simulink model "SISO_simulink_model"  (R2022a)
settings: Solver=VariableStepAuto  StartTime=0.0  StopTime=3  RelTol=1e-3
model workspace (MAT data in the model file):
  C = Simulink.Parameter
  C.Value = 525.1
  C.DataType = 'auto'
  C.Complexity = 'real'
  C.Dimensions = [1 1]
  D = Simulink.Parameter
  D.Value = 0.6069
  D.Description = 'Damping EFE'
  D.DataType = 'auto'
  D.Complexity = 'real'
  D.Dimensions = [1 1]
  I = Simulink.Parameter
  I.Value = 0.075809
  I.Description = 'Inertia EFE'
  I.DataType = 'auto'
  I.Complexity = 'real'
  I.Dimensions = [1 1]
  I_inv = Simulink.Parameter
  I_inv.Value = 13.191045918
  I_inv.DataType = 'auto'
  I_inv.Complexity = 'real'
  I_inv.Dimensions = [1 1]
  K = Simulink.Parameter
  K.Value = 8.67
  K.DataType = 'auto'
  K.Complexity = 'real'
  K.Dimensions = [1 1]
  M = Simulink.Parameter
  M.Value = 0.045754
  M.Description = 'Moment arm of Biceps Long Head on EFE.'
  M.DataType = 'auto'
  M.Complexity = 'real'
  M.Dimensions = [1 1]
  T_1 = Simulink.Parameter
  T_1.Value = 0.03
  T_1.DataType = 'auto'
  T_1.Complexity = 'real'
  T_1.Dimensions = [1 1]
  T_2 = Simulink.Parameter
  T_2.Value = 0.04
  T_2.DataType = 'auto'
  T_2.Complexity = 'real'
  T_2.Dimensions = [1 1]
values from neighbouring files (symbols this model uses):
  C = 525.1    [SISO_Model.m]
  D = 0.6069    [SISO_Model.m]
  I_inv = inv(I)    [SISO_Model.m]
  K = 8.67    [SISO_Model.m]
  M = 0.045754    [SISO_Model.m]
  T_1 = 0.03    [SISO_Model.m]
  T_2 = 0.04    [SISO_Model.m]
settings Model: Creator=ians  LastModifiedBy=ians

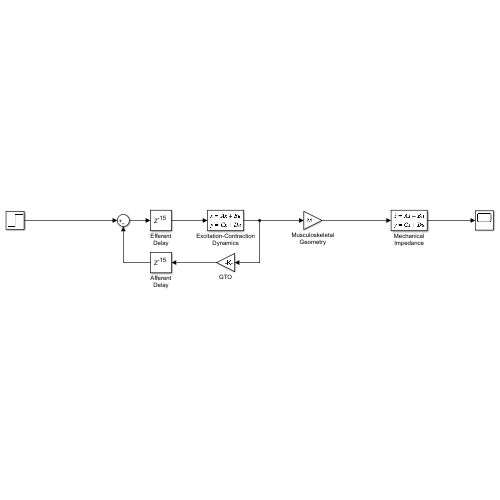
[thumbnail: Simulink's stored preview of the top-level diagram]
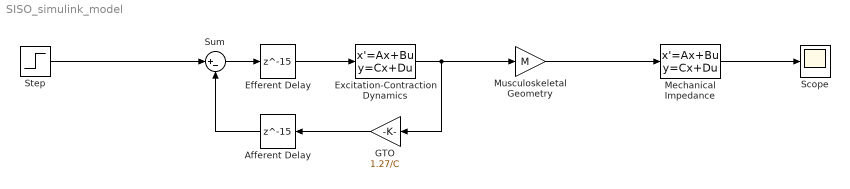
== system SISO_simulink_model ==
  Afferent Delay : Delay  DelayLength=15
  Efferent Delay : Delay  DelayLength=15
  Excitation-Contraction Dynamics : StateSpace  A=[0, 1; -1/(T_1*T_2), -(T_1+T_2)/(T_1*T_2)]  B=[0; C/(T_1*T_2)]  C=[1, 0]  D=0  InitialCondition=0
  GTO : Gain  Gain=1.27/C
  Mechanical Impedance : StateSpace  A=[0, 1; -I_inv*K, -I_inv*D]  B=[0; I_inv]  C=[1, 0]  D=0  InitialCondition=0  ParameterTunability=Optimized  ContinuousStateAttributes='q'
  Musculoskeletal Geometry : Gain  Gain=M
  Scope : Scope
  Step : Step  SampleTime=0.001
  Sum : Sum  Inputs=|+-
  wires:
  Excitation-Contraction Dynamics/1 -> Musculoskeletal Geometry/1, GTO/1
  GTO/1 -> Afferent Delay/1
  Efferent Delay/1 -> Excitation-Contraction Dynamics/1
  Sum/1 -> Efferent Delay/1
  Afferent Delay/1 -> Sum/2
  Mechanical Impedance/1 -> Scope/1
  Step/1 -> Sum/1
  Musculoskeletal Geometry/1 -> Mechanical Impedance/1
